simulink model "delay_track_fshift_sim"  (R2019a)
settings: Solver=VariableStepAuto  StartTime=0.0  StopTime=500000 / (fs_ghz * 1e9)  RelTol=1e-3
undefined symbols (not defined in the file or in its folder): fdesignblkfcn, fs_ghz, gcbh
libraries: dspmtrx3 x5, dspxfrm3 x2, simulink x1
(part 3 of 7)

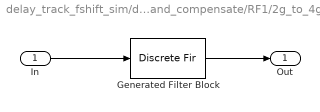
== system delay_track_fshift_sim/delay_and_compensate/RF1/2g_to_4g_filt ==
  In : Inport
  Generated Filter Block : DiscreteFir  Tag=BlockMethodSubSystem  Coefficients=[2.93722382866788096e-05 3.41459391652129034e-05 3.77128110868576443e-05 3.99224737036247014e-05 4.06853079430514713e-05 3.99767906724050358e-05 3.78385630665936822e-05 3.43761762884411585e-05 2.97536321530244167e-05 2.41850044819596572e-05 1.79235799255994288e-05 1.12490869892622225e-05 4.4536819092569802e-06 -2.17257546056165917e-06 -8.35599694025994471e-06 -1.38525483000206094e-05 -1.84594484756624878e-05 -2.20244865077465419e-05 -2.44525796905669946e-05 -2.57092444736974581e-05 -2.58208171862182267e-05 -2.48714358220079919e-05 -2.29969676250314427e-05 -2.03762307559743188e-05 -1.7220003129447142e-05 -1.37584297927058172e-05 -1.02275255841993233e-05 -6.85551762427440588e-06 -3.84977981433300826e-06 -1.38507846695198298e-06 4.06223847654850621e-07 1.44146638159053655e-06 1.69208708312454467e-06 1.18487405565268557e-06 -6.06728885075140407e-19 -1.7340549530134312e-06 -3.84841475535380876e-06 -6.14411864234574767e-06 -8.40426300697009752e-06 -1.04073009831605586e-05 -1.1940758993427882e-05 -1.2814601750957214e-05 -1.28734911642698022e-05 -1.20072397436402085e-05 -1.01588527025680601e-05 -7.32968014996432518e-06 -3.58135490934933877e-06 9.65635577496104344e-07 6.13671231869329652e-06 1.17110896017580304e-05 1.74323961589531137e-05 2.30214944323852813e-05 2.81908346649924015e-05 3.26595902087329341e-05 3.61687699202395182e-05 3.84954958141815645e-05 3.94656699944219444e-05 3.89643326804979111e-05 3.69431290294147452e-05 3.3424450490399247e-05 2.85019889302292616e-05 2.23376296739663695e-05 1.51548029794998283e-05 7.22860200377775612e-06 -1.12685108638701611e-06 -9.57315993364699036e-06 -1.77637820032781818e-05 -2.53607041599212844e-05 -3.20508056170196547e-05 -3.75610589674782409e-05 -4.16717760723184981e-05 -4.42272041116535385e-05 -4.51429130909003571e-05 -4.44095825104338107e-05 -4.20929830419749398e-05 -3.83301489863486426e-05 -3.33219383980320111e-05 -2.73223693070855402e-05 -2.06252921501967482e-05 -1.35491010431840891e-05 -6.42029209833677532e-06 4.43260242918632263e-07 6.74842152024941793e-06 1.22414540126946882e-05 1.67204329906863005e-05 2.00447629304407976e-05 2.21412895596018245e-05 2.30066868003525849e-05 2.27059989416843563e-05 2.13674269413795351e-05 1.91736524025005777e-05 1.6350182399041591e-05 1.31513625879524334e-05 9.84483588726477108e-06 6.69531216783360987e-06 3.94855584700627589e-06 1.81649042570595134e-06 4.64261964345005076e-07 0 4.67869756437844547e-07 1.84483124954039099e-06 4.04131848336743271e-06 6.90583619204581518e-06 1.02332541468990554e-05 1.37763717431228871e-05 1.72601397835483777e-05 2.03977723989025532e-05 2.29078685600185678e-05 2.45315962057293983e-05 2.50489766973744071e-05 2.4293344450284416e-05 2.21631446876514145e-05 1.86303670412677299e-05 1.37450873455755861e-05 7.63579537217579106e-06 5.05411612779898964e-07 -7.37687046457391485e-06 -1.56875515410801046e-05 -2.40640261138680043e-05 -3.21222548229339687e-05 -3.94760053700459601e-05 -4.57566608275759219e-05 -5.06325497962671397e-05 -5.38267642754433636e-05 -5.51324982274634226e-05 -5.44250596151723447e-05 -5.16698752611954059e-05 -4.692601273682605e-05 -4.03449760055476272e-05 -3.21647794987187251e-05 -2.26995555169551265e-05 -1.23251889114210383e-05 -1.46168796015643012e-06 9.44682055156931247e-06 1.99534507556481698e-05 2.9630170436965972e-05 3.80885441271285865e-05 4.49985216569913921e-05 5.01042836026001172e-05 5.32363049823407768e-05 5.43189944560376156e-05 5.33734979743676863e-05 5.05155111447766445e-05 4.59482099543780285e-05 3.99506706982889623e-05 3.28623928846142444e-05 2.50647502743081311e-05 1.69603634074791312e-05 8.95150254720619725e-06 1.41868628553046558e-06 -5.2993653954292894e-06 -1.09233341595465557e-05 -1.52475019605648257e-05 -1.8149766833923053e-05 -1.95969229982492455e-05 -1.96449097134478252e-05 -1.84340085374496237e-05 -1.61792468798566039e-05 -1.31565319194244876e-05 -9.68527840579672232e-06 -6.10849329641758076e-06 -2.77142833562077375e-06 1.31357454865854822e-18 1.91980067254066973e-06 ...(+56375 chars)]  InputProcessing=Columns as channels (frame based)
  Out : Outport
  wires:
  In/1 -> Generated Filter Block/1
  Generated Filter Block/1 -> Out/1
